simulink model "lab3_2"  (R2020a)
settings: Solver=VariableStepAuto  StartTime=0.0  StopTime=10.0  RelTol=1e-3
settings Model: Creator=huang  LastModifiedBy=huang

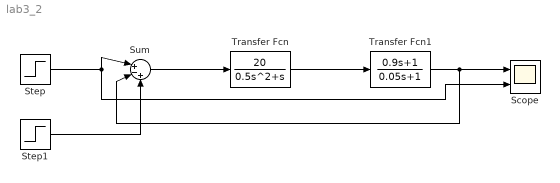
== system lab3_2 ==
  Scope : Scope  NumInputPorts=2
  Step : Step  Time=0  SampleTime=0
  Step1 : Step  Time=2  After=-1  SampleTime=0
  Sum : Sum  Inputs=|+-+
  Transfer Fcn : TransferFcn  Numerator=[20]  Denominator=[0.5 1 0]
  Transfer Fcn1 : TransferFcn  Numerator=[0.9 1]  Denominator=[0.05 1]
  wires:
  Sum/1 -> Transfer Fcn/1
  Transfer Fcn/1 -> Transfer Fcn1/1
  Transfer Fcn1/1 -> Sum/2, Scope/1
  Step/1 -> Scope/2, Sum/1
  Step1/1 -> Sum/3
